simulink model "vehicleArrivedDataStatus"  (R2021a)
settings: Solver=VariableStepAuto  StartTime=0.0  StopTime=10.0  RelTol=1e-3
undefined symbols (not defined in the file): DiscIntNeverNeededParam
libraries: simulink x1
settings Model: Creator=Utkarsh Anand  LastModifiedBy=Utkarsh Anand
settings DataIOCC: SaveOutput=off  SaveTime=off

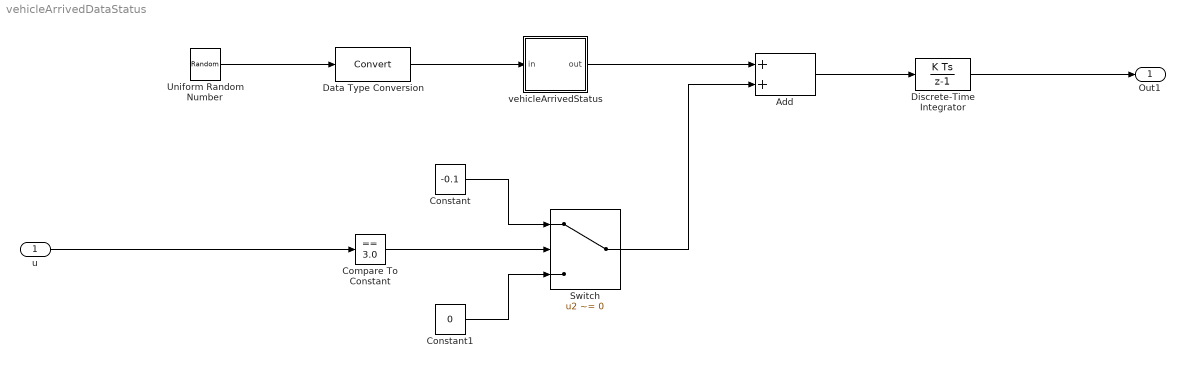
== system vehicleArrivedDataStatus ==
  u : Inport  OutDataTypeStr=double  PortDimensions=1  SampleTime=[0,1]
  Add : Sum
  Compare To Constant : simulink/Logic and Bit Operations/Compare To Constant  relop===  const=3.0  OutDataTypeStr=boolean
  Constant : Constant  Value=-0.1
  Constant1 : Constant  Value=0
  Data Type Conversion : DataTypeConversion
  Discrete-Time Integrator : DiscreteIntegrator  SampleTime=-1  LimitOutput=on  LowerSaturationLimit=0  ICPrevOutput=DiscIntNeverNeededParam  ICPrevScaledInput=DiscIntNeverNeededParam
  Switch : Switch  Criteria=u2 ~= 0
  Uniform Random Number : UniformRandomNumber  Minimum=0  Maximum=100  Seed=177836  SampleTime=0
  vehicleArrivedStatus : Stateflow chart  TreatAsAtomicUnit=on
  Out1 : Outport  OutDataTypeStr=double  PortDimensions=1  SampleTime=[0.20000000000000001,0]
  wires:
  Constant1/1 -> Switch/3
  Uniform Random Number/1 -> Data Type Conversion/1
  Compare To Constant/1 -> Switch/2
  vehicleArrivedStatus/1(out) -> Add/1
  Switch/1 -> Add/2
  Add/1 -> Discrete-Time Integrator/1
  Data Type Conversion/1 -> vehicleArrivedStatus/1(in)
  Constant/1 -> Switch/1
  u/1 -> Compare To Constant/1
  Discrete-Time Integrator/1 -> Out1/1

== stateflow chart vehicleArrivedDataStatus/vehicleArrivedStatus ==
  (default) -> (junction 7) : {out = in > 98;}
  data: in input int8; out output double
